simulink model "five_bar"  (R2024a)
settings: Solver=ode3  StartTime=0  StopTime=Tstop  FixedStep=Tsim  RelTol=1e-3  EnableMultiTasking=on
values from neighbouring files (symbols this model uses):
  Bm = 1e-6    (= 1e-06)    [five_bar_init.m]
  K = K_start    [five_bar_init.m]
  Koef_m = 2.1    [five_bar_init.m]
  Koef_w = 24    [five_bar_init.m]
  Mext = 16    [five_bar_init.m]
  Mext_start = 5    [five_bar_init.m]
  Mext_stop = 7.5    [five_bar_init.m]
  psi_f = 1-Ra    (= 0.925)    [five_bar_init.m]
  Ra = 0.075    [DC_model_init.m]    (also in five_bar_init.m)
  Ta = 20e-3    (= 0.02)    [DC_model_init.m]    (also in five_bar_init.m = 0.001)
  Tm = 0.5    [DC_model_init.m]    (also in five_bar_init.m)
  Tsim = 10e-3    (= 0.01)    [DC_model_init.m]    (also in five_bar_init.m = 0.001)
  w = [1, 4, 1.5]    [five_bar_init.m]
  x_ref = -50e-3    (= -0.05)    [five_bar_init.m]
  x_start = 50e-3    (= 0.05)    [five_bar_init.m]
  y_ref = 20e-3    (= 0.02)    [five_bar_init.m]
  y_start = 20e-3    (= 0.02)    [five_bar_init.m]
libraries: slpidlib x2
settings Model: Creator=Pop  LastModifiedBy=lazar
settings SolverCC: AlgebraicLoopSolver=TrustRegion
settings DataIOCC: LimitDataPoints=on  SaveFormat=Array  ReturnWorkspaceOutputs=off
settings OptimizationCC: LifeSpan=inf
settings DebuggingCC: AlgebraicLoopMsg=none  SolverPrmCheckMsg=warning  MultiTaskRateTransMsg=warning  UnconnectedInputMsg=warning  UnconnectedOutputMsg=warning  UnconnectedLineMsg=warning  SFUnexpectedBacktrackingDiag=warning  SFNoUnconditionalDefaultTransitionDiag=warning  SFExecutionAtInitializationDiag=none  ArithmeticOperatorsInVariantConditions=warning
settings HardwareCC: ProdBitPerPointer=32  ProdBitPerSizeT=32  ProdBitPerPtrDiffT=32  ProdLargestAtomicFloat=None  ProdIntDivRoundTo=Undefined  ProdEndianess=Unspecified  ProdWordSize=32  ProdHWDeviceType=32-bit Generic
settings ModelReferenceCC: PropagateSignalLabelsOutOfModel=off
settings SFSimCC: SimUseLocalCustomCode=off  CustomCodeUndefinedFunction=UseInterfaceOnly
settings RTWCC: RTWUseLocalCustomCode=off  GPUComputeCapability=3.5
settings CodeAppCC: StateflowObjectComments=on
settings GRTTargetCC: TargetLangStandard=C89/C90 (ANSI)
settings ConfigComp: CovMetricSettings=dw  CovSaveCumulativeToWorkspaceVar=on  CovSaveSingleToWorkspaceVar=on  CovExternalEMLEnable=off  CovSFcnEnable=off

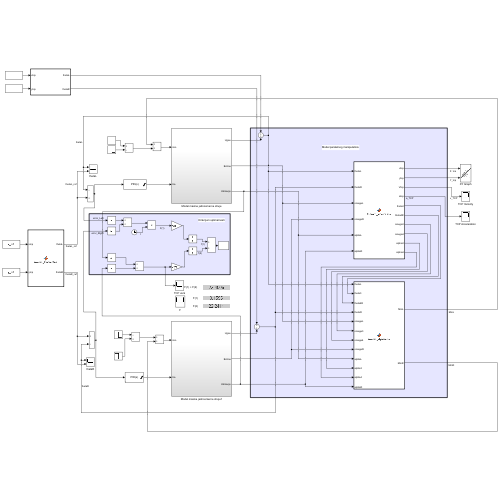
[thumbnail: Simulink's stored preview of the top-level diagram]
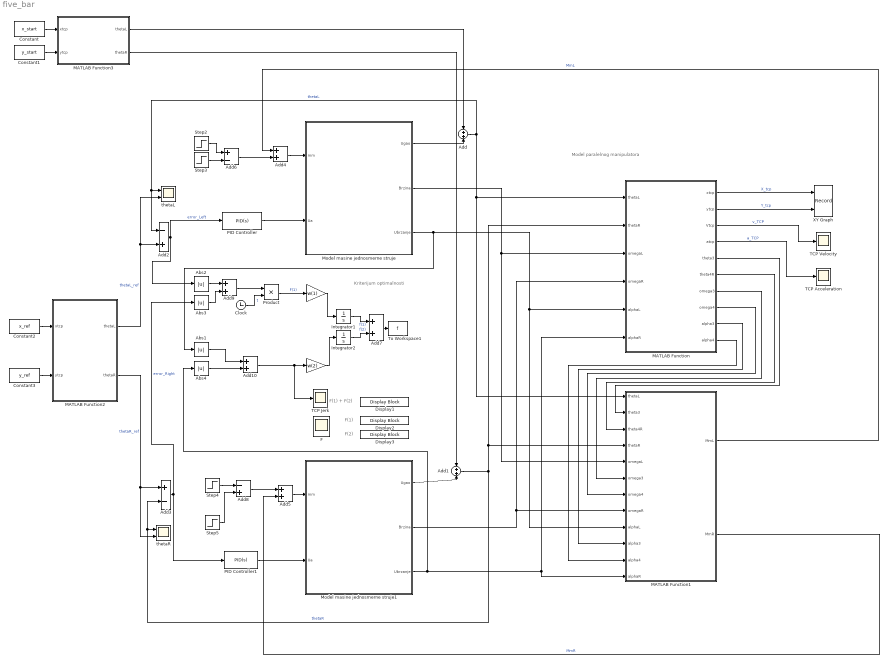
== system five_bar ==
  note: F(2)
  note: F(1)
  note: Kriterijum optimalnosti
  note: Model paralelnog manipulatora
  note: F(1) + F(2)
  "    " : Gain  Gain=w(2)  SampleTime=Tsim
  "     " : Gain  Gain=w(1)  SampleTime=Tsim
  Abs{1..4} (4 alike) : Abs  SaturateOnIntegerOverflow=off
  Add{,1,4..5,7,9..10} (7 alike) : Sum
  Add2 : Sum  Inputs=-+
  Add3 : Sum  Inputs=+-
  Add6 : Sum  Inputs=+-
  Add8 : Sum  Inputs=-+
  Clock : Clock
  Constant : Constant  Value=x_start
  Constant1 : Constant  Value=y_start
  Constant2 : Constant  Value=x_ref
  Constant3 : Constant  Value=y_ref
  Display1 : DisplayBlock  LabelPosition=Hide  Transparency=1
  Display2 : DisplayBlock  LabelPosition=Hide  Transparency=1
  Display3 : DisplayBlock  LabelPosition=Hide  Transparency=1
  F : Scope
      settings: Floating=on
  Integrator1 : Integrator
  Integrator2 : Integrator
  MATLAB Function : MATLAB Function  TreatAsAtomicUnit=on
  MATLAB Function1 : MATLAB Function  TreatAsAtomicUnit=on
  MATLAB Function2 : MATLAB Function  TreatAsAtomicUnit=on
  MATLAB Function3 : MATLAB Function  TreatAsAtomicUnit=on
  Model masine jednosmerne struje : Subsystem
  Model masine jednosmerne struje1 : Subsystem
  PID Controller : slpidlib/PID Controller  Controller=PID  Form=Parallel  TimeDomain=Continuous-time  UseExternalTs=off  SampleTime=-1  IntegratorMethod=Forward Euler  FilterMethod=Forward Euler  ControllerParametersSource=internal  P=K(1)  I=K(2)  UseKiTs=off  D=K(3)  UseExternalDerivativeSource=off  N=100  UseFilter=on  TunerSelectOption=Transfer Function Based (PID Tuner App)  InitialConditionSource=internal  InitialConditionForIntegrator=0  InitialConditionForFilter=0  DifferentiatorICPrevScaledInput=0  ExternalReset=none  TrackingMode=off  Kt=1  LimitOutput=on  SatLimitsSource=internal  UpperSaturationLimit=1  LowerSaturationLimit=-1  LinearizeAsGain=on  AntiWindupMode=clamping  Kb=1  LimitIntegrator=off  UpperIntegratorSaturationLimit=inf  LowerIntegratorSaturationLimit=-inf  POutMin=[]  POutMax=[]  IOutMin=[]  IOutMax=[]  DOutMin=[]  DOutMax=[]  NOutMin=[]  NOutMax=[]  SumOutMin=[]  SumOutMax=[]  SaturationOutMin=[]  SaturationOutMax=[]  PParamMin=[]  PParamMax=[]  IParamMin=[]  IParamMax=[]  DParamMin=[]  DParamMax=[]  NParamMin=[]  NParamMax=[]  KbParamMin=[]  KbParamMax=[]  KtParamMin=[]  KtParamMax=[]  KbOutMin=[]  KbOutMax=[]  KtOutMin=[]  KtOutMax=[]  IntegratorOutMin=[]  IntegratorOutMax=[]  FilterOutMin=[]  FilterOutMax=[]  SumI1OutMin=[]  SumI1OutMax=[]  SumI2OutMin=[]  SumI2OutMax=[]  SumI3OutMin=[]  SumI3OutMax=[]  SumI4OutMin=[]  SumI4OutMax=[]  SumDOutMin=[]  SumDOutMax=[]  DifferentiatorOutMin=[]  DifferentiatorOutMax=[]  FilterDiffOutCoefMin=[]  FilterDiffOutCoefMax=[]  ReciprocalOutMin=[]  ReciprocalOutMax=[]  SumDenOutMin=[]  SumDenOutMax=[]  SumNumOutMin=[]  SumNumOutMax=[]  DivideOutMin=[]  DivideOutMax=[]  UdiffTsProdOutMin=[]  UdiffTsProdOutMax=[]  NTsProdOutMin=[]  NTsProdOutMax=[]  UintegralTsProdOutMin=[]  UintegralTsProdOutMax=[]  UngainTsProdOutMin=[]  UngainTsProdOutMax=[]  ClampingZeroOutDataTypeStr=Inherit: Inherit via back propagation  ClampingZeroOutMin=[]  ClampingZeroOutMax=[]  FilterDenConstantOutDataTypeStr=Inherit: Inherit via back propagation  FilterDenConstantOutMin=[]  FilterDenConstantOutMax=[]  PCopyOutDataTypeStr=Inherit: Inherit via back propagation  PCopyOutMin=[]  PCopyOutMax=[]  NCopyOutDataTypeStr=Inherit: Inherit via back propagation  NCopyOutMin=[]  NCopyOutMax=[]  IntegratorContinuousStateAttributes=''  IntegratorStateMustResolveToSignalObject=off  IntegratorRTWStateStorageClass=Auto  FilterContinuousStateAttributes=''  FilterStateMustResolveToSignalObject=off  FilterRTWStateStorageClass=Auto  ParallelPVariant=InternalParameters  IdealPVariant=Disabled  IVariant=InternalParameters  DVariant=InternalParameters  IntegratorVariant=Continuous  SatVariant=Enabled  AWVariant=ContClampingParallel  PCopyVariant=Disabled  TRVariant=Disabled  FdbkBlocksVariant=Forward  IdealPFdbkVariant=Disabled  SatFdbkVariant=Disabled  DerivativeFilterVariant=ContFilter  NVariant=InternalParameters  NCopyVariant=Disabled  FilterICVariant=InternalICsFilter  IntegratorICVariant=InternalICs  ExternalResetVariant=Disabled  TRSumVariant=Passthrough  SumFdbkVariant=Disabled  SumVariant=Sum_PID  TsampFilterVariant=InternalTs  TsampNgainVariant=Passthrough  TsampIntegralVariant=Disabled_SignalSpec  ExternalSaturationOutDataTypeStr=Inherit: Same as second input  DerivativeSourceVariant=ErrorSignal
  PID Controller1 : slpidlib/PID Controller  Controller=PID  Form=Parallel  TimeDomain=Continuous-time  UseExternalTs=off  SampleTime=-1  IntegratorMethod=Forward Euler  FilterMethod=Forward Euler  ControllerParametersSource=internal  P=K(1)  I=K(2)  UseKiTs=off  D=K(3)  UseExternalDerivativeSource=off  N=100  UseFilter=on  TunerSelectOption=Transfer Function Based (PID Tuner App)  InitialConditionSource=internal  InitialConditionForIntegrator=0  InitialConditionForFilter=0  DifferentiatorICPrevScaledInput=0  ExternalReset=none  TrackingMode=off  Kt=1  LimitOutput=on  SatLimitsSource=internal  UpperSaturationLimit=1  LowerSaturationLimit=-1  LinearizeAsGain=on  AntiWindupMode=clamping  Kb=1  LimitIntegrator=off  UpperIntegratorSaturationLimit=inf  LowerIntegratorSaturationLimit=-inf  POutMin=[]  POutMax=[]  IOutMin=[]  IOutMax=[]  DOutMin=[]  DOutMax=[]  NOutMin=[]  NOutMax=[]  SumOutMin=[]  SumOutMax=[]  SaturationOutMin=[]  SaturationOutMax=[]  PParamMin=[]  PParamMax=[]  IParamMin=[]  IParamMax=[]  DParamMin=[]  DParamMax=[]  NParamMin=[]  NParamMax=[]  KbParamMin=[]  KbParamMax=[]  KtParamMin=[]  KtParamMax=[]  KbOutMin=[]  KbOutMax=[]  KtOutMin=[]  KtOutMax=[]  IntegratorOutMin=[]  IntegratorOutMax=[]  FilterOutMin=[]  FilterOutMax=[]  SumI1OutMin=[]  SumI1OutMax=[]  SumI2OutMin=[]  SumI2OutMax=[]  SumI3OutMin=[]  SumI3OutMax=[]  SumI4OutMin=[]  SumI4OutMax=[]  SumDOutMin=[]  SumDOutMax=[]  DifferentiatorOutMin=[]  DifferentiatorOutMax=[]  FilterDiffOutCoefMin=[]  FilterDiffOutCoefMax=[]  ReciprocalOutMin=[]  ReciprocalOutMax=[]  SumDenOutMin=[]  SumDenOutMax=[]  SumNumOutMin=[]  SumNumOutMax=[]  DivideOutMin=[]  DivideOutMax=[]  UdiffTsProdOutMin=[]  UdiffTsProdOutMax=[]  NTsProdOutMin=[]  NTsProdOutMax=[]  UintegralTsProdOutMin=[]  UintegralTsProdOutMax=[]  UngainTsProdOutMin=[]  UngainTsProdOutMax=[]  ClampingZeroOutDataTypeStr=Inherit: Inherit via back propagation  ClampingZeroOutMin=[]  ClampingZeroOutMax=[]  FilterDenConstantOutDataTypeStr=Inherit: Inherit via back propagation  FilterDenConstantOutMin=[]  FilterDenConstantOutMax=[]  PCopyOutDataTypeStr=Inherit: Inherit via back propagation  PCopyOutMin=[]  PCopyOutMax=[]  NCopyOutDataTypeStr=Inherit: Inherit via back propagation  NCopyOutMin=[]  NCopyOutMax=[]  IntegratorContinuousStateAttributes=''  IntegratorStateMustResolveToSignalObject=off  IntegratorRTWStateStorageClass=Auto  FilterContinuousStateAttributes=''  FilterStateMustResolveToSignalObject=off  FilterRTWStateStorageClass=Auto  ParallelPVariant=InternalParameters  IdealPVariant=Disabled  IVariant=InternalParameters  DVariant=InternalParameters  IntegratorVariant=Continuous  SatVariant=Enabled  AWVariant=ContClampingParallel  PCopyVariant=Disabled  TRVariant=Disabled  FdbkBlocksVariant=Forward  IdealPFdbkVariant=Disabled  SatFdbkVariant=Disabled  DerivativeFilterVariant=ContFilter  NVariant=InternalParameters  NCopyVariant=Disabled  FilterICVariant=InternalICsFilter  IntegratorICVariant=InternalICs  ExternalResetVariant=Disabled  TRSumVariant=Passthrough  SumFdbkVariant=Disabled  SumVariant=Sum_PID  TsampFilterVariant=InternalTs  TsampNgainVariant=Passthrough  TsampIntegralVariant=Disabled_SignalSpec  ExternalSaturationOutDataTypeStr=Inherit: Same as second input  DerivativeSourceVariant=ErrorSignal
  Product : Product
  Step2 : Step  Time=Mext_start  After=Mext  SampleTime=0
  Step3 : Step  Time=Mext_stop  After=Mext  SampleTime=0
  Step4 : Step  Time=Mext_start  After=Mext  SampleTime=0
  Step5 : Step  Time=Mext_stop  After=Mext  SampleTime=0
  TCP Acceleration : Scope
  TCP Jerk : Scope
  TCP Velocity : Scope
  To Workspace1 : ToWorkspace  VariableName=f  SampleTime=-1
      settings: Save2DSignal=2-D array (concatenate along first dimension)
  XY Graph : Record  FileSettingsInternal="{\"entries\":[{\"content\":{\"excelSettings\":{\"content\":{},\"type\":\"Streamout.ExcelSettings\"}},\"type\":\"Streamout.FileSettingStorage\",\"uuid\":\"\"}],\"packageUris\":[\"http:\\/\\/schema.mathworks.com\\/mf0\\/streamout_blocks\\/R2020a\"],\"version\":\"1.0\"}"  Layout=[1 1]  SignalsInternal="{\"entries\":[{\"content\":{\"signals\":[{\"content\":{\"blockPath\":[],\"dimensions\":[1],\"domain\":\"\",\"lineColor\":\"#a2142f\",\"plots\":[ 1 ],\"port\":1,\"sid\":[\"\"],\"signalID\":1,\"signalName\":\"X_tcp\"},\"type\":\"RecordBlkView.Signal\",\"uuid\":\"\"},{\"content\":{\"blockPath\":[],\"dimensions\":[1],\"domain\":\"\",\"lineColor\":\"#139fff\",\"plots\":[ 1 ],\"port\":2,\"sid\":[\"\"],\"signalID\":2,\"signalName\":\"Y_tcp\"},\"type\":\"RecordBlkView.Signal\",\"uuid\":\"\"}]},\"type\":\"RecordBlkView.InputSignals\",\"uuid\":\"\"}],\"packageUris\":[\"http:\\/\\/schema.mathworks.com\\/mf0\\/streamout_blocks\\/R2020a\"],\"version\":\"1.0\"}"  VisualizationBindings="{\"xyplotplugin\":{\"info\":[{\"series\":[{\"bindingParametersList\":[{\"parameter\":\"X-Axis\",\"signalID\":1,\"signalName\":\"X_tcp\"},{\"parameter\":\"Y-Axis\",\"signalID\":2,\"signalName\":\"Y_tcp\"}],\"seriesID\":0}],\"subplotID\":1}]}}"  CompatibilityTag=XY
  thetaL : Scope  NumInputPorts=2
  thetaR : Scope  NumInputPorts=2
  wires:
  MATLAB Function/1(xtcp) -> XY Graph/1  "X_tcp"
  MATLAB Function/2(ytcp) -> XY Graph/2  "Y_tcp"
  MATLAB Function1/1(MmL) -> Add4/1  "MmL"
  MATLAB Function1/2(MmR) -> Add5/2  "MmR"
  Add/1 -> MATLAB Function1/1(thetaL), MATLAB Function/1(thetaL), thetaL/1, Add2/1  "thetaL"
  Add1/1 -> Add3/2, thetaR/1, MATLAB Function/2(thetaR), MATLAB Function1/4(thetaR)  "thetaR"
  Model masine jednosmerne struje/2(Brzina) -> MATLAB Function1/5(omegaL), MATLAB Function/3(omegaL)
  Model masine jednosmerne struje1/2(Brzina) -> MATLAB Function/4(omegaR), MATLAB Function1/8(omegaR)
  Model masine jednosmerne struje/3(Ubrzanje) -> Abs1/1, MATLAB Function/5(alphaL), MATLAB Function1/9(alphaL)
  Model masine jednosmerne struje1/3(Ubrzanje) -> Abs4/1, MATLAB Function1/12(alphaR), MATLAB Function/6(alphaR)
  MATLAB Function/5(theta3) -> MATLAB Function1/2(theta3)
  MATLAB Function/6(theta4R) -> MATLAB Function1/3(theta4R)
  MATLAB Function/7(omega3) -> MATLAB Function1/6(omega3)
  MATLAB Function/8(omega4) -> MATLAB Function1/7(omega4)
  MATLAB Function/9(alpha3) -> MATLAB Function1/10(alpha3)
  MATLAB Function/10(alpha4) -> MATLAB Function1/11(alpha4)
  Model masine jednosmerne struje/1(Ugao) -> Add/2
  MATLAB Function3/1(thetaL) -> Add/1
  Model masine jednosmerne struje1/1(Ugao) -> Add1/2
  Constant2/1 -> MATLAB Function2/1(xtcp)
  Constant3/1 -> MATLAB Function2/2(ytcp)
  MATLAB Function2/1(thetaL) -> Add2/2, thetaL/2  "thetaL_ref"
  MATLAB Function2/2(thetaR) -> thetaR/2, Add3/1  "thetaR_ref"
  Add2/1 -> PID Controller/1, Abs2/1  "error_Left"
  Add3/1 -> PID Controller1/1, Abs3/1  "error_Right"
  Constant1/1 -> MATLAB Function3/2(ytcp)
  Constant/1 -> MATLAB Function3/1(xtcp)
  MATLAB Function3/2(thetaR) -> Add1/1
  Abs3/1 -> Add9/2
  PID Controller1/1 -> Model masine jednosmerne struje1/2(Ua)
  PID Controller/1 -> Model masine jednosmerne struje/2(Ua)
  Add4/1 -> Model masine jednosmerne struje/1(mm)
  Step2/1 -> Add6/1
  Add5/1 -> Model masine jednosmerne struje1/1(mm)
  Step3/1 -> Add6/2
  Step4/1 -> Add8/1
  Step5/1 -> Add8/2
  Abs2/1 -> Add9/1
  Add6/1 -> Add4/2
  Add8/1 -> Add5/1
  "     "/1 -> Integrator1/1
  MATLAB Function/3(Vtcp) -> TCP Velocity/1  "v_TCP"
  MATLAB Function/4(atcp) -> TCP Acceleration/1  "a_TCP"
  "    "/1 -> Integrator2/1
  Add7/1 -> To Workspace1/1
  Product/1 -> "     "/1  "F(1)"
  Clock/1 -> Product/2  "t"
  Add9/1 -> Product/1
  Integrator2/1 -> Add7/2  "f(2)"
  Integrator1/1 -> Add7/1  "f(1)"
  Add10/1 -> "    "/1, TCP Jerk/1
  Abs1/1 -> Add10/1
  Abs4/1 -> Add10/2

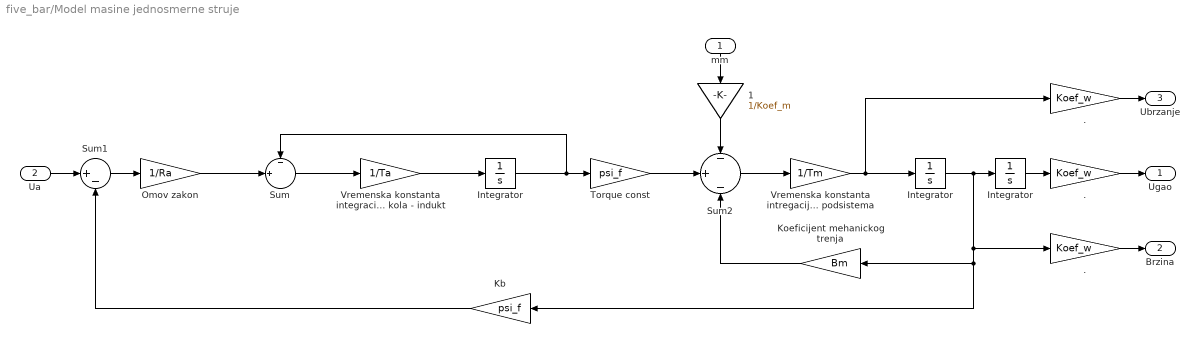
== system five_bar/Model masine jednosmerne struje ==
  mm : Inport
  Ua : Inport  Port=2
  "   Integrator   " : Integrator
  "  Integrator  " : Integrator
  " ." : Gain  Gain=Koef_w  SampleTime=Tsim
  " 1" : Gain  Gain=1/Koef_m  SampleTime=Tsim
  . : Gain  Gain=Koef_w  SampleTime=Tsim
  ". " : Gain  Gain=Koef_w  SampleTime=Tsim
  Integrator : Integrator
  Kb : Gain  Gain=psi_f  SampleTime=Tsim
  Koeficijent mehanickog trenja : Gain  Gain=Bm  SampleTime=Tsim
  Omov zakon : Gain  Gain=1/Ra  SampleTime=Tsim
  Sum : Sum  Inputs=-|+||  SampleTime=Tsim
  Sum1 : Sum  Inputs=|+-  SampleTime=Tsim
  Sum2 : Sum  Inputs=-||+||-  SampleTime=Tsim
  Torque const : Gain  Gain=psi_f  SampleTime=Tsim
  Vremenska konstanta integracije rotorskog kola - indukt : Gain  Gain=1/Ta  SampleTime=Tsim
  Vremenska konstanta intregacije mehanickog podsistema : Gain  Gain=1/Tm  SampleTime=Tsim
  Ugao : Outport
  Brzina : Outport  Port=2
  Ubrzanje : Outport  Port=3
  wires:
  Ua/1 -> Sum1/1
  Kb/1 -> Sum1/2
  ". "/1 -> Brzina/1
  "  Integrator  "/1 -> "   Integrator   "/1, Kb/1, Koeficijent mehanickog trenja/1, ". "/1
  ./1 -> Ubrzanje/1
  "   Integrator   "/1 -> " ."/1
  Sum2/1 -> Vremenska konstanta intregacije mehanickog podsistema/1
  mm/1 -> " 1"/1
  Sum/1 -> Vremenska konstanta integracije rotorskog kola - indukt/1
  Vremenska konstanta integracije rotorskog kola - indukt/1 -> Integrator/1
  Koeficijent mehanickog trenja/1 -> Sum2/3
  Integrator/1 -> Sum/1, Torque const/1
  " ."/1 -> Ugao/1
  Torque const/1 -> Sum2/2
  Sum1/1 -> Omov zakon/1
  Omov zakon/1 -> Sum/2
  Vremenska konstanta intregacije mehanickog podsistema/1 -> "  Integrator  "/1, ./1
  " 1"/1 -> Sum2/1

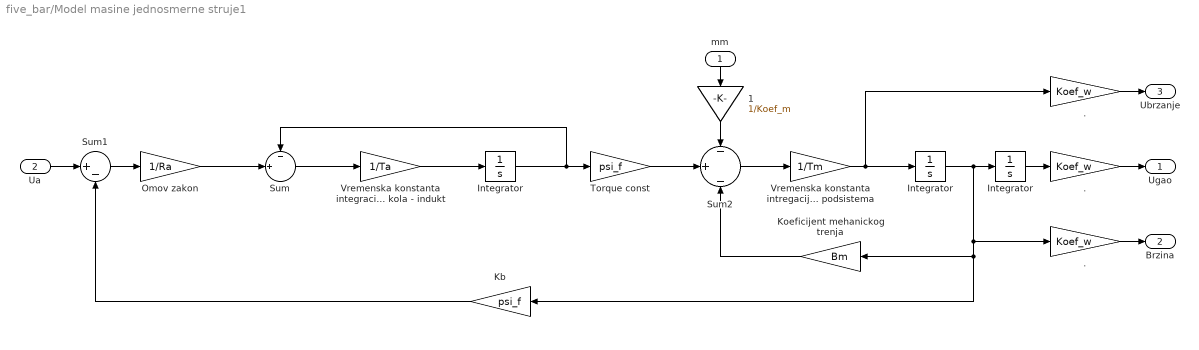
== system five_bar/Model masine jednosmerne struje1 ==
  mm : Inport
  Ua : Inport  Port=2
  "   Integrator   " : Integrator
  "  Integrator  " : Integrator
  " ." : Gain  Gain=Koef_w  SampleTime=Tsim
  " 1" : Gain  Gain=1/Koef_m  SampleTime=Tsim
  . : Gain  Gain=Koef_w  SampleTime=Tsim
  ". " : Gain  Gain=Koef_w  SampleTime=Tsim
  Integrator : Integrator
  Kb : Gain  Gain=psi_f  SampleTime=Tsim
  Koeficijent mehanickog trenja : Gain  Gain=Bm  SampleTime=Tsim
  Omov zakon : Gain  Gain=1/Ra  SampleTime=Tsim
  Sum : Sum  Inputs=-|+||  SampleTime=Tsim
  Sum1 : Sum  Inputs=|+-  SampleTime=Tsim
  Sum2 : Sum  Inputs=-||+||-  SampleTime=Tsim
  Torque const : Gain  Gain=psi_f  SampleTime=Tsim
  Vremenska konstanta integracije rotorskog kola - indukt : Gain  Gain=1/Ta  SampleTime=Tsim
  Vremenska konstanta intregacije mehanickog podsistema : Gain  Gain=1/Tm  SampleTime=Tsim
  Ugao : Outport
  Brzina : Outport  Port=2
  Ubrzanje : Outport  Port=3
  wires:
  Ua/1 -> Sum1/1
  Kb/1 -> Sum1/2
  ". "/1 -> Brzina/1
  "  Integrator  "/1 -> "   Integrator   "/1, Kb/1, Koeficijent mehanickog trenja/1, ". "/1
  ./1 -> Ubrzanje/1
  "   Integrator   "/1 -> " ."/1
  Sum2/1 -> Vremenska konstanta intregacije mehanickog podsistema/1
  mm/1 -> " 1"/1
  Sum/1 -> Vremenska konstanta integracije rotorskog kola - indukt/1
  Vremenska konstanta integracije rotorskog kola - indukt/1 -> Integrator/1
  Koeficijent mehanickog trenja/1 -> Sum2/3
  Integrator/1 -> Sum/1, Torque const/1
  " ."/1 -> Ugao/1
  Torque const/1 -> Sum2/2
  Sum1/1 -> Omov zakon/1
  Omov zakon/1 -> Sum/2
  Vremenska konstanta intregacije mehanickog podsistema/1 -> "  Integrator  "/1, ./1
  " 1"/1 -> Sum2/1

== matlab function five_bar/MATLAB Function1 ==
  data: thetaL input; MmL output; theta3 input; theta4R input; thetaR input; omegaL input; omega3 input; omega4 input; omegaR input; alphaL input; alpha3 input; alpha4 input; alphaR input; MmR output
function [MmL, MmR] = inverse_dynamics(thetaL, theta3, theta4R, thetaR, omegaL, omega3, omega4, omegaR, alphaL, alpha3, alpha4, alphaR)
    [~, P, D, mP, mD, JsP, JsD] = get_params();
    
    m2 = mP;
    m5 = mP;
    m3 = mD;
    m4 = mD;
    Js2 = JsP;
    Js5 = JsP;
    Js3 = JsD;
    Js4 = JsD;
    
    as2x = - P/2 * omegaL^2 * cos(thetaL) - P/2 * alphaL * sin(thetaL);
    as2y = - P/2 * omegaL^2 * sin(thetaL) + P/2 * alphaL * cos(thetaL);
    as3x = - P * omegaL^2 * cos(thetaL) - P * alphaL * sin(thetaL) - D/2 * omega3^2 * cos(theta3) - D/2 * alpha3 * sin(theta3);
    as3y = - P * omegaL^2 * sin(thetaL) + P * alphaL * cos(thetaL) - D/2 * omega3^2 * sin(theta3) + D/2 * alpha3 * cos(theta3);
    as4x = - P * omegaR^2 * cos(thetaR) - P * alphaR * sin(thetaR) - D/2 * omega4^2 * cos(theta4R) - D/2 * alpha4 * sin(theta4R);
    as4y = - P * omegaR^2 * sin(thetaR) + P * alphaR * cos(thetaR) - D/2 * omega4^2 * sin(theta4R) + D/2 * alpha4 * cos(theta4R);
    as5x = - P/2 * omegaR^2 * cos(thetaR) - P/2 * alphaR * sin(thetaR);
    as5y = - P/2 * omegaR^2 * sin(thetaR) + P/2 * alphaR * cos(thetaR);

    A_d = [ 1, 0, 0, 1, 0, 0, 0, 0, 0, 0, 0, 0;
            0, 1, 0, 0, 1, 0, 0, 0, 0, 0, 0, 0;
            P/2*sin(thetaL), -P/2*cos(thetaL), 1, -P/2*sin(thetaL), P/2*cos(thetaL), 0, 0, 0, 0, 0, 0, 0;
            0, 0, 0, -1, 0, 1, 0, 0, 0, 0, 0, 0;
            0, 0, 0, 0, -1, 0, 1, 0, 0, 0, 0, 0;
            0, 0, 0, -D/2*sin(theta3), D/2*cos(theta3), -D/2*sin(theta3), D/2*cos(theta3), 0, 0, 0, 0, 0;
            0, 0, 0, 0, 0, -1, 0, 1, 0, 0, 0, 0;
            0, 0, 0, 0, 0, 0, -1, 0, 1, 0, 0, 0;
            0, 0, 0, 0, 0, D/2*sin(theta4R), -D/2*cos(theta4R), D/2*sin(theta4R), -D/2*cos(theta4R), 0, 0, 0;
            0, 0, 0, 0, 0, 0, 0, -1, 0, 1, 0, 0;
            0, 0, 0, 0, 0, 0, 0, 0, -1, 0, 1, 0;
            0, 0, 0, 0, 0, 0, 0, -P/2*sin(thetaR), P/2*cos(thetaR), -P/2*sin(thetaR), P/2*cos(thetaR), 1
          ];
    B_d = [ m2 * as2x;
            m2 * as2y;
            Js2 * alphaL;
            m3 * as3x;
            m3 * as3y;
            Js3 * alpha3;
            m4 * as4x;
            m4 * as4y;
            Js4 * alpha4;
            m5 * as5x;
            m5 * as5y;
            Js5 * alphaR
          ];
    D = A_d \ B_d;
    MmL = D(3);
    MmR = D(12);
end

== matlab function five_bar/MATLAB Function ==
  data: thetaL input; xtcp output; thetaR input; omegaL input; omegaR input; alphaL input; alphaR input; ytcp output; Vtcp output; atcp output; theta3 output; theta4R output; omega3 output; omega4 output; alpha3 output; alpha4 output
function [xtcp, ytcp, Vtcp, atcp, theta3, theta4R, omega3, omega4, alpha3, alpha4] = forward_kinematics(thetaL, thetaR, omegaL, omegaR, alphaL, alphaR)
    [L,P,D] = get_params();

    xA = -L/2 + P * cos(thetaL);
    yA = P * sin(thetaL);
    xB = L/2 + P * cos(thetaR);
    yB = P * sin(thetaR);

    A = (xB - xA) / D;
    B = (yB - yA) / D;
    C = (A*A + B*B) / 2;
    A1 = (xA - xB) / D;
    B1 = (yA - yB) / D;

    theta4R = 2*atan2(-B-sqrt(A*A+B*B-C*C), C-A);
    theta3 = 2*atan2(-B1+sqrt(A1*A1+B1*B1-C*C), C-A1);
    xtcp = xA + D*cos(theta3);
    ytcp = yA + D*sin(theta3);

    % Velocities
    A_v = [ -1, 0, - D*sin(theta3), 0;
            -1, 0, 0, - D*sin(theta4R);
            0, 1, - D*cos(theta3), 0;
            0, 1, 0, - D*cos(theta4R)
            ];
    B_v = [ omegaL*P*sin(thetaL);
            omegaR*P*sin(thetaR);
            omegaL*P*cos(thetaL);
            omegaR*P*cos(thetaR)
          ];
    V = A_v \ B_v;
    Vxtcp = V(1);
    Vytcp = V(2);
    omega3 = V(3);
    omega4 = V(4);
    Vtcp = sqrt(Vxtcp^2+Vytcp^2);

    % Accelerations
    A_a = [ 1, 0, D*sin(theta3), 0;
            1, 0, 0, D*sin(theta4R);
            0, 1, -D*cos(theta3), 0;
            0, 1, 0, -D*cos(theta4R)
            ];
    B_a = [ -P*sin(thetaL)*alphaL - P*cos(thetaL)*omegaL^2 - D*cos(theta3)*omega3^2;
            -P*sin(thetaR)*alphaR - P*cos(thetaR)*omegaR^2 - D*cos(theta4R)*omega4^2;
            P*cos(thetaL)*alphaL - P*sin(thetaL)*omegaL^2 - D*sin(theta3)*omega3^2;
            P*cos(thetaR)*alphaR - P*sin(thetaR)*omegaR^2 - D*sin(theta4R)*omega4^2
          ];
    A = A_a \ B_a;
    axtcp = A(1);
    aytcp = A(2);
    alpha3 = A(3);
    alpha4 = A(4);
    atcp = sqrt(axtcp^2+aytcp^2);
end

== matlab function five_bar/MATLAB Function2 ==
  data: xtcp input; thetaL output; ytcp input; thetaR output
function [thetaL, thetaR] = inverse_kinematics(xtcp,ytcp)
    [L,P,D] = get_params();

    C1 = ((xtcp + L/2)^2 + ytcp^2 + P^2 - D^2) / (2*ytcp*P);
    C2 = (xtcp + L/2) / ytcp;
    C3 = ((xtcp - L/2)^2 + ytcp^2 + P^2 - D^2) / (2*ytcp*P);
    C4 = (xtcp - L/2) / ytcp;

    thetaL = 2*atan2(1+sqrt(1-C1*C1+C2*C2), C1+C2);
    thetaR = 2*atan2(1-sqrt(1-C3*C3+C4*C4), C3+C4);

    thetaL = wrapTo2Pi(thetaL);
    thetaR = wrapToPi(thetaR);
end

== matlab function five_bar/MATLAB Function3 ==
  data: xtcp input; thetaL output; ytcp input; thetaR output
function [thetaL, thetaR] = inverse_kinematics(xtcp,ytcp)
    [L,P,D] = get_params();

    C1 = ((xtcp + L/2)^2 + ytcp^2 + P^2 - D^2) / (2*ytcp*P);
    C2 = (xtcp + L/2) / ytcp;
    C3 = ((xtcp - L/2)^2 + ytcp^2 + P^2 - D^2) / (2*ytcp*P);
    C4 = (xtcp - L/2) / ytcp;

    thetaL = 2*atan2(1+sqrt(1-C1*C1+C2*C2), C1+C2);
    thetaR = 2*atan2(1-sqrt(1-C3*C3+C4*C4), C3+C4);

    thetaL = wrapTo2Pi(thetaL);
    thetaR = wrapToPi(thetaR);
end
